simulink model "A2_SMART_Traffic_Automation_System_Outcome1"  (R2024b)
settings: Solver=VariableStepAuto  StartTime=0.0  StopTime=inf  RelTol=1e-3
settings Model: NumberOfSteps=2  Creator=User  LastModifiedBy=User

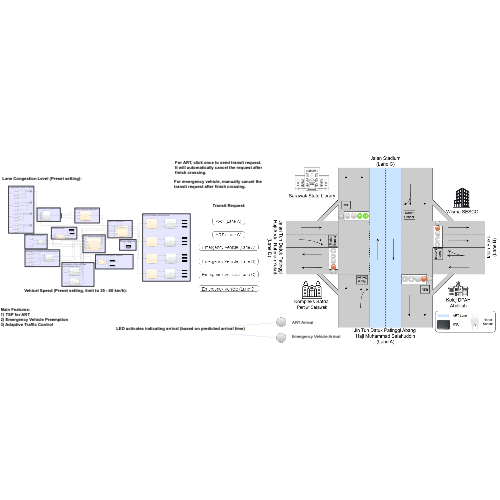
[thumbnail: Simulink's stored preview of the top-level diagram]
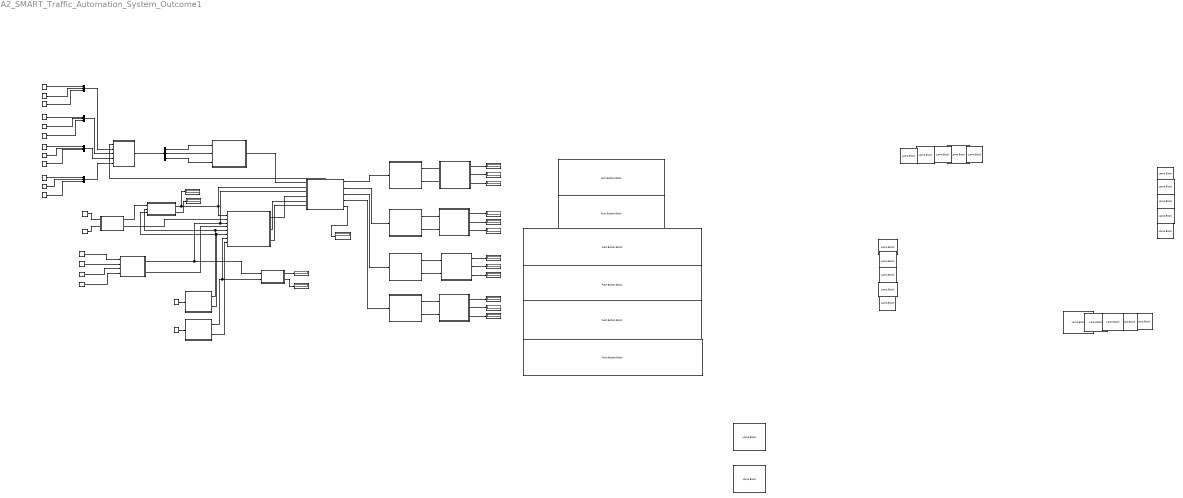
== system A2_SMART_Traffic_Automation_System_Outcome1 ==
  note: Transit Request:
  note: Lane A
  note: Congestion Level of Lanes
  note: Classification of Congestion Level
  note: Green Interval Selection
  note: Traffic Controller
  note: ART Transit Request
  note: Emergency Vehicle Transit Request
  note: Arrival of ART
  note: TSP Request Handling
  note: Arrival of Emergency Vehicle
  note: Calculation of Arrival Time
      | and Crossing Time
  note: Flash Signal
  note: Light Controller and Decoder
  note: ART Arrival
  note: Emergency Vehicle Arrival
  note: Lane B
  note: Lane C
  note: Lane D
  note: For ART, click once to send transit request. It will automatically cancel the request after finish crossing.
      |
      | For emergency vehicle, manually cancel the transit request after finish crossing.
  note: LED activates indicating arrival (based on predicted arrival time)
  note: Lane Congestion Level (Preset setting):
  note: Main Features:
      | 1) TSP for ART
      | 2) Emergency Vehicle Preemption
      | 3) Adaptive Traffic Control
  note: Vehicel Speed (Preset setting, limit to 35 - 80 km/h):
  ART Arrival : Display
  ART Transit Request : Display
  Calculation of ART Arrival Time and Crossing Time : Subsystem
  Calculation of Emergency Vehicle Arrival Time and Crossing Time : Subsystem
  Chart : Stateflow chart  TreatAsAtomicUnit=on
      settings: PortSchema="{\"entries\":[{\"content\":{\"sides\":[{\"content\":{\"connectorIds\":[\"In6\",\"In8\",\"In5\",\"In7\",\"In1\",\"In3\",\"In2\",\"In4\"]},\"type\":\"ConnectorPlacement.EquallySpacedRectSide\",\"uuid\":\"3b8b5f25-9f42-4404-a7ab-9a14576ba9bc\"},{\"content\":{\"connectorIds\":[\"Out3\",\"Out1\",\"Out2\"],\"side\":\"RIGHT\"},\"type\":\"ConnectorPlacement.EquallySpacedRectSide\",\"uuid\":\"4c53b1e2-c9f4-4e0d-a7f8-e259704f49e5\"},{\"content\":{\"side\":\"TOP\"},\"type\":\"ConnectorPlacement.EquallySpacedRectSide\",\"uuid\":\"8c5bac8d-90e8-4795-8438-ca30e0de2823\"}]},\"type\":\"ConnectorPlacement.EquallySpacedConnector\",\"uuid\":\"481cd6a2-dbd3-4912-a805-bd25a54799f5\"}],\"packageUris\":[\"http://schema.mathworks.com/mf0/Connector/R2020b\"],\"version\":\"1.0\"}"
  Chart1 : Stateflow chart  TreatAsAtomicUnit=on
  Chart2 : Stateflow chart  TreatAsAtomicUnit=on
      settings: PortSchema="{\"entries\":[{\"content\":{\"sides\":[{\"content\":{\"connectorIds\":[\"In1\",\"In2\"]},\"type\":\"ConnectorPlacement.EquallySpacedRectSide\",\"uuid\":\"14131ada-69d8-4c61-8553-b2a1dbc3d743\"},{\"content\":{\"connectorIds\":[\"Out2\",\"Out1\"],\"side\":\"RIGHT\"},\"type\":\"ConnectorPlacement.EquallySpacedRectSide\",\"uuid\":\"91a87b04-e272-4077-aa78-32a12e8e289e\"},{\"content\":{\"side\":\"TOP\"},\"type\":\"ConnectorPlacement.EquallySpacedRectSide\",\"uuid\":\"3c65f825-8df3-4d64-be65-7907849d7437\"}]},\"type\":\"ConnectorPlacement.EquallySpacedConnector\",\"uuid\":\"a2eb85a8-e87b-481d-83e5-614a6250d93d\"}],\"packageUris\":[\"http://schema.mathworks.com/mf0/Connector/R2020b\"],\"version\":\"1.0\"}"
  Decoder (Lane A) : Subsystem
  Decoder (Lane B) : Subsystem
  Decoder (Lane C) : Subsystem
  Decoder (Lane D) : Subsystem
  Demux : Demux  Outputs=3
  Display{,1..11} (12 alike) : Display
  Emergency Vehicle Arrival : Display
  Emergency Vehicle Transit Request : Display
  Flash : Display
  High Congestion A : Constant  Value=0
  High Congestion B : Constant  Value=0
  High Congestion C : Constant
  High Congestion D : Constant  Value=0
  Lamp{,1,12,16..17,20..23,26..27,29,31..32} (14 alike) : LampBlock  LabelPosition=Hide
  Lamp13 : LampBlock  LabelPosition=Hide  Icon=Custom  CustomIcon=data:image/svg+xml;base64,PD94bWwgdmVyc2lvbj0iMS4wIiBlbmNvZGluZz0idXRmLTgiPz4NCg0KPCEtLSBVcGxvYWRlZCB0bzogU1ZHIFJlcG8sIHd3dy5zdmdyZXBvLmNvbSwgR2VuZXJhdG9yOiBTVkcgUmVwbyBNaXhlciBUb29scyAtLT4KPHN2ZyBmaWxsPSIjMDAwMDAwIiBoZWlnaHQ9IjgwMHB4IiB3aWR0aD0iODAwcHgiIHZlcnNpb249IjEuMSIgaWQ9Ikljb25zIiB4bWxucz0iaHR0cDovL3d3dy53My5vcmcvMjAwMC9zdmciIHhtbG5zOnhsaW5rPSJodHRwOi8vd3d3LnczLm9yZy8xOTk5L3hsaW5rIiANCgkgdmlld0JveD0iMCAwIDMyIDMyIiB4bWw6c3BhY2U9InByZXNlcnZlIj4NCjxwYXRoIGQ9Ik0xNiwyQzguMywyLDIsOC4zLDIsMTZzNi4zLDE0LDE0LDE0czE0LTYuMywxNC0xNFMyMy43LDIsMTYsMnogTTIwLjcsMTUuN0MyMC41LDE1LjksMjAuMywxNiwyMCwxNnMtMC41LTAuMS0wLjctMC4zDQoJTDE3LDEzLjRWMjJjMCwwLjYtMC40LDEtMSwxcy0xLTAuNC0xLTF2LTguNmwtMi4zLDIuM2MtMC40LDAuNC0xLDAuNC0xLjQsMHMtMC40LTEsMC0xLjRsNC00YzAuMS0wLjEsMC4yLTAuMiwwLjMtMC4yDQoJYzAuMi0wLjEsMC41LTAuMSwwLjgsMGMwLjEsMC4xLDAuMiwwLjEsMC4zLDAuMmw0LDRDMjEuMSwxNC43LDIxLjEsMTUuMywyMC43LDE1Ljd6Ii8+DQo8L3N2Zz4=
  Lamp14 : LampBlock  LabelPosition=Hide  Icon=Custom  CustomIcon=data:image/svg+xml;base64,PD94bWwgdmVyc2lvbj0iMS4wIiBlbmNvZGluZz0iaXNvLTg4NTktMSI/Pg0KPCEtLSBVcGxvYWRlZCB0bzogU1ZHIFJlcG8sIHd3dy5zdmdyZXBvLmNvbSwgR2VuZXJhdG9yOiBTVkcgUmVwbyBNaXhlciBUb29scyAtLT4NCjxzdmcgaGVpZ2h0PSI4MDBweCIgd2lkdGg9IjgwMHB4IiB2ZXJzaW9uPSIxLjEiIGlkPSJDYXBhXzEiIHhtbG5zPSJodHRwOi8vd3d3LnczLm9yZy8yMDAwL3N2ZyIgeG1sbnM6eGxpbms9Imh0dHA6Ly93d3cudzMub3JnLzE5OTkveGxpbmsiIA0KCSB2aWV3Qm94PSIwIDAgMjYuOTI3IDI2LjkyNyIgeG1sOnNwYWNlPSJwcmVzZXJ2ZSI+DQo8Zz4NCgk8ZyBpZD0iYzE5NF9hcnJvdyI+DQoJCTxwYXRoIHN0eWxlPSJmaWxsOiMwMzAxMDQ7IiBkPSJNMTMuNDY0LDAuMDAyQzYuMDI3LDAuMDAyLDAsNi4wMjcsMCwxMy40NjRjMCw3LjQzNSw2LjAyNywxMy40NjIsMTMuNDY0LDEzLjQ2Mg0KCQkJYzcuNDMyLDAsMTMuNDYzLTYuMDI3LDEzLjQ2My0xMy40NjJDMjYuOTI4LDYuMDI3LDIwLjg5NiwwLjAwMiwxMy40NjQsMC4wMDJ6IE0yMi44MTYsMTUuMzAybC02LjM1NSw2LjM1NA0KCQkJYy0wLjgyNiwwLjgyOC0yLjEyMSwwLjg2Ny0yLjg5NSwwLjA5NGMtMC43NzItMC43NzMtMC43MzItMi4wNjgsMC4wOTQtMi44OTNsMy4wNC0zLjA0Mkg1LjQ0N2MtMS4wOTcsMC0xLjk4Mi0wLjg4OC0xLjk4NC0xLjk4MQ0KCQkJYzAtMS4wOTQsMC44ODctMS45OCwxLjk4NC0xLjk4aDExLjMxMUwxMy43MDIsOC44Yy0wLjgxMi0wLjgxNC0wLjg0Ny0yLjEwMy0wLjA3LTIuODc1YzAuNzczLTAuNzcyLDIuMDU4LTAuNzQxLDIuODcxLDAuMDczDQoJCQlsNi4yNzEsNi4yNjhjMC4wMjcsMC4wMjcsMC4wNDcsMC4wNjIsMC4wNywwLjA4OGMwLjAyMywwLjAyLDAuMDQ3LDAuMDMzLDAuMDY2LDAuMDU0QzIzLjY4NCwxMy4xNzcsMjMuNjQzLDE0LjQ3NCwyMi44MTYsMTUuMzAyeg0KCQkJIi8+DQoJPC9nPg0KPC9nPg0KPC9zdmc+
  Lamp18 : LampBlock  LabelPosition=Hide  Icon=Custom  CustomIcon=data:image/svg+xml;base64,PD94bWwgdmVyc2lvbj0iMS4wIiBlbmNvZGluZz0iVVRGLTgiIHN0YW5kYWxvbmU9Im5vIj8+DQo8IS0tIFVwbG9hZGVkIHRvOiBTVkcgUmVwbywgd3d3LnN2Z3JlcG8uY29tLCBHZW5lcmF0b3I6IFNWRyBSZXBvIE1peGVyIFRvb2xzIC0tPg0KPHN2ZyB3aWR0aD0iODAwcHgiIGhlaWdodD0iODAwcHgiIHZpZXdCb3g9IjAgMCAzMiAzMiIgdmVyc2lvbj0iMS4xIiB4bWxucz0iaHR0cDovL3d3dy53My5vcmcvMjAwMC9zdmciIHhtbG5zOnhsaW5rPSJodHRwOi8vd3d3LnczLm9yZy8xOTk5L3hsaW5rIiB4bWxuczpza2V0Y2g9Imh0dHA6Ly93d3cuYm9oZW1pYW5jb2RpbmcuY29tL3NrZXRjaC9ucyI+DQogICAgDQogICAgPHRpdGxlPmFycm93LXJpZ2h0LWNpcmNsZTwvdGl0bGU+DQogICAgPGRlc2M+Q3JlYXRlZCB3aXRoIFNrZXRjaCBCZXRhLjwvZGVzYz4NCiAgICA8ZGVmcz4NCg0KPC9kZWZzPg0KICAgIDxnIGlkPSJQYWdlLTEiIHN0cm9rZT0ibm9uZSIgc3Ryb2tlLXdpZHRoPSIxIiBmaWxsPSJub25lIiBmaWxsLXJ1bGU9ImV2ZW5vZGQiIHNrZXRjaDp0eXBlPSJNU1BhZ2UiPg0KICAgICAgICA8ZyBpZD0iSWNvbi1TZXQtRmlsbGVkIiBza2V0Y2g6dHlwZT0iTVNMYXllckdyb3VwIiB0cmFuc2Zvcm09InRyYW5zbGF0ZSgtMzEwLjAwMDAwMCwgLTEwODkuMDAwMDAwKSIgZmlsbD0iIzAwMDAwMCI+DQogICAgICAgICAgICA8cGF0aCBkPSJNMzMyLjUzNSwxMTA1Ljg4IEwzMjYuODc5LDExMTEuNTQgQzMyNi40ODgsMTExMS45MyAzMjUuODU1LDExMTEuOTMgMzI1LjQ2NSwxMTExLjU0IEMzMjUuMDc0LDExMTEuMTUgMzI1LjA3NCwxMTEwLjUxIDMyNS40NjUsMTExMC4xMiBMMzI5LjU4NiwxMTA2IEwzMTksMTEwNiBDMzE4LjQ0NywxMTA2IDMxOCwxMTA1LjU1IDMxOCwxMTA1IEMzMTgsMTEwNC40NSAzMTguNDQ3LDExMDQgMzE5LDExMDQgTDMyOS41ODYsMTEwNCBMMzI1LjQ2NSwxMDk5Ljg4IEMzMjUuMDc0LDEwOTkuNDkgMzI1LjA3NCwxMDk4Ljg2IDMyNS40NjUsMTA5OC40NiBDMzI1Ljg1NSwxMDk4LjA3IDMyNi40ODgsMTA5OC4wNyAzMjYuODc5LDEwOTguNDYgTDMzMi41MzUsMTEwNC4xMiBDMzMyLjc3NSwxMTA0LjM2IDMzMi44NSwxMTA0LjY5IDMzMi43OTUsMTEwNSBDMzMyLjg1LDExMDUuMzEgMzMyLjc3NSwxMTA1LjY0IDMzMi41MzUsMTEwNS44OCBMMzMyLjUzNSwxMTA1Ljg4IFogTTMyNiwxMDg5IEMzMTcuMTYzLDEwODkgMzEwLDEwOTYuMTYgMzEwLDExMDUgQzMxMCwxMTEzLjg0IDMxNy4xNjMsMTEyMSAzMjYsMTEyMSBDMzM0LjgzNywxMTIxIDM0MiwxMTEzLjg0IDM0MiwxMTA1IEMzNDIsMTA5Ni4xNiAzMzQuODM3LDEwODkgMzI2LDEwODkgTDMyNiwxMDg5IFoiIGlkPSJhcnJvdy1yaWdodC1jaXJjbGUiIHNrZXRjaDp0eXBlPSJNU1NoYXBlR3JvdXAiPg0KDQo8L3BhdGg+DQogICAgICAgIDwvZz4NCiAgICA8L2c+DQo8L3N2Zz4=
  Lamp19 : LampBlock  LabelPosition=Hide  Icon=Custom  CustomIcon=data:image/svg+xml;base64,PD94bWwgdmVyc2lvbj0iMS4wIiBlbmNvZGluZz0idXRmLTgiPz4KDTwhLS0gVXBsb2FkZWQgdG86IFNWRyBSZXBvLCB3d3cuc3ZncmVwby5jb20sIEdlbmVyYXRvcjogU1ZHIFJlcG8gTWl4ZXIgVG9vbHMgLS0+Cjxzdmcgd2lkdGg9IjgwMHB4IiBoZWlnaHQ9IjgwMHB4IiB2aWV3Qm94PSIwIDAgMjQgMjQiIHhtbG5zPSJodHRwOi8vd3d3LnczLm9yZy8yMDAwL3N2ZyI+CiAgICA8Zz4KICAgICAgICA8cGF0aCBmaWxsPSJub25lIiBkPSJNMCAwaDI0djI0SDB6Ii8+CiAgICAgICAgPHBhdGggZD0iTTEyIDJjNS41MiAwIDEwIDQuNDggMTAgMTBzLTQuNDggMTAtMTAgMTBTMiAxNy41MiAyIDEyIDYuNDggMiAxMiAyem0wIDlWOGwtNCA0IDQgNHYtM2g0di0yaC00eiIvPgogICAgPC9nPgo8L3N2Zz4=
  Lamp24 : LampBlock  LabelPosition=Hide  Icon=Custom  CustomIcon=data:image/svg+xml;base64,PD94bWwgdmVyc2lvbj0iMS4wIiBlbmNvZGluZz0iaXNvLTg4NTktMSI/Pg0KPCEtLSBVcGxvYWRlZCB0bzogU1ZHIFJlcG8sIHd3dy5zdmdyZXBvLmNvbSwgR2VuZXJhdG9yOiBTVkcgUmVwbyBNaXhlciBUb29scyAtLT4NCjwhRE9DVFlQRSBzdmcgUFVCTElDICItLy9XM0MvL0RURCBTVkcgMS4xLy9FTiIgImh0dHA6Ly93d3cudzMub3JnL0dyYXBoaWNzL1NWRy8xLjEvRFREL3N2ZzExLmR0ZCI+DQo8c3ZnIGZpbGw9IiMwMDAwMDAiIHZlcnNpb249IjEuMSIgaWQ9IkNhcGFfMSIgeG1sbnM9Imh0dHA6Ly93d3cudzMub3JnLzIwMDAvc3ZnIiB4bWxuczp4bGluaz0iaHR0cDovL3d3dy53My5vcmcvMTk5OS94bGluayIgDQoJIHdpZHRoPSI4MDBweCIgaGVpZ2h0PSI4MDBweCIgdmlld0JveD0iMCAwIDQwIDQwIiB4bWw6c3BhY2U9InByZXNlcnZlIj4NCjxnPg0KCTxwYXRoIGQ9Ik0yMCwwQzguOTczLDAsMCw4Ljk3MywwLDIwYzAsMTEuMDI3LDguOTczLDIwLDIwLDIwYzExLjAyNywwLDIwLTguOTczLDIwLTIwQzQwLDguOTczLDMxLjAyNywwLDIwLDB6IE0yOC4wMTgsMTkuNzUyDQoJCWMtMC40NTEsMC41MzEtMS4wOTQsMC44MDUtMS43MzgsMC44MDVjLTAuNTIxLDAtMS4wNDctMC4xNzktMS40NzctMC41NDNsLTIuNTIxLTIuMTQxdjkuMTg2YzAsMS4yNi0xLjAyMSwyLjI4LTIuMjgxLDIuMjgNCgkJYy0xLjI2LDAtMi4yODEtMS4wMjEtMi4yODEtMi4yOHYtOS4xODZsLTIuNTIxLDIuMTQxYy0wLjk2LDAuODE2LTIuNCwwLjY5OC0zLjIxNi0wLjI2MmMtMC44MTYtMC45NjEtMC42OTgtMi40LDAuMjYyLTMuMjE2DQoJCWw2LjI3OS01LjMzM2MwLjg1Mi0wLjcyMywyLjEwMi0wLjcyMywyLjk1NSwwbDYuMjc4LDUuMzMzQzI4LjcxNiwxNy4zNTIsMjguODM0LDE4Ljc5MSwyOC4wMTgsMTkuNzUyeiIvPg0KPC9nPg0KPC9zdmc+
  Lamp25 : LampBlock  LabelPosition=Hide  Icon=Custom  CustomIcon=data:image/svg+xml;base64,PD94bWwgdmVyc2lvbj0iMS4wIiBlbmNvZGluZz0iaXNvLTg4NTktMSI/Pg0KPCEtLSBVcGxvYWRlZCB0bzogU1ZHIFJlcG8sIHd3dy5zdmdyZXBvLmNvbSwgR2VuZXJhdG9yOiBTVkcgUmVwbyBNaXhlciBUb29scyAtLT4NCjwhRE9DVFlQRSBzdmcgUFVCTElDICItLy9XM0MvL0RURCBTVkcgMS4xLy9FTiIgImh0dHA6Ly93d3cudzMub3JnL0dyYXBoaWNzL1NWRy8xLjEvRFREL3N2ZzExLmR0ZCI+DQo8c3ZnIGZpbGw9IiMwMDAwMDAiIHZlcnNpb249IjEuMSIgaWQ9IkNhcGFfMSIgeG1sbnM9Imh0dHA6Ly93d3cudzMub3JnLzIwMDAvc3ZnIiB4bWxuczp4bGluaz0iaHR0cDovL3d3dy53My5vcmcvMTk5OS94bGluayIgDQoJIHdpZHRoPSI4MDBweCIgaGVpZ2h0PSI4MDBweCIgdmlld0JveD0iMCAwIDQwIDQwIiB4bWw6c3BhY2U9InByZXNlcnZlIj4NCjxnPg0KCTxwYXRoIGQ9Ik0yMCwwQzguOTczLDAsMCw4Ljk3MywwLDIwYzAsMTEuMDI3LDguOTczLDIwLDIwLDIwYzExLjAyNywwLDIwLTguOTczLDIwLTIwQzQwLDguOTczLDMxLjAyNywwLDIwLDB6IE0yNy43NTYsMjMuNDY1DQoJCWwtNi4yNzksNS4zMzJDMjEuMDUxLDI5LjE1OCwyMC41MjUsMjkuMzQsMjAsMjkuMzRjLTAuNTI2LDAtMS4wNTItMC4xODItMS40NzgtMC41NDNsLTYuMjc5LTUuMzMyDQoJCWMtMC45NTktMC44MTYtMS4wNzctMi4yNTYtMC4yNjItMy4yMTdjMC44MTUtMC45NTksMi4yNTUtMS4wNzgsMy4yMTYtMC4yNjJsMi41MjEsMi4xNDF2LTkuMTg2YzAtMS4yNiwxLjAyMS0yLjI4MSwyLjI4Mi0yLjI4MQ0KCQljMS4yNiwwLDIuMjgxLDEuMDIxLDIuMjgxLDIuMjgxdjkuMTg2bDIuNTIxLTIuMTQxYzAuOTYyLTAuODE0LDIuNDAxLTAuNjk3LDMuMjE4LDAuMjYyDQoJCUMyOC44MzQsMjEuMjA5LDI4LjcxNiwyMi42NDgsMjcuNzU2LDIzLjQ2NXoiLz4NCjwvZz4NCjwvc3ZnPg==
  Lamp28 : LampBlock  LabelPosition=Hide  Icon=Custom  CustomIcon=data:image/svg+xml;base64,PD94bWwgdmVyc2lvbj0iMS4wIiBlbmNvZGluZz0idXRmLTgiPz4KDTwhLS0gVXBsb2FkZWQgdG86IFNWRyBSZXBvLCB3d3cuc3ZncmVwby5jb20sIEdlbmVyYXRvcjogU1ZHIFJlcG8gTWl4ZXIgVG9vbHMgLS0+Cjxzdmcgd2lkdGg9IjgwMHB4IiBoZWlnaHQ9IjgwMHB4IiB2aWV3Qm94PSIwIDAgMjQgMjQiIHhtbG5zPSJodHRwOi8vd3d3LnczLm9yZy8yMDAwL3N2ZyI+CiAgICA8Zz4KICAgICAgICA8cGF0aCBmaWxsPSJub25lIiBkPSJNMCAwaDI0djI0SDB6Ii8+CiAgICAgICAgPHBhdGggZD0iTTEyIDJjNS41MiAwIDEwIDQuNDggMTAgMTBzLTQuNDggMTAtMTAgMTBTMiAxNy41MiAyIDEyIDYuNDggMiAxMiAyem0wIDlWOGwtNCA0IDQgNHYtM2g0di0yaC00eiIvPgogICAgPC9nPgo8L3N2Zz4=
  Lamp30 : LampBlock  LabelPosition=Hide  Icon=Custom  CustomIcon=data:image/svg+xml;base64,PD94bWwgdmVyc2lvbj0iMS4wIiBlbmNvZGluZz0iaXNvLTg4NTktMSI/Pg0KPCEtLSBVcGxvYWRlZCB0bzogU1ZHIFJlcG8sIHd3dy5zdmdyZXBvLmNvbSwgR2VuZXJhdG9yOiBTVkcgUmVwbyBNaXhlciBUb29scyAtLT4NCjwhRE9DVFlQRSBzdmcgUFVCTElDICItLy9XM0MvL0RURCBTVkcgMS4xLy9FTiIgImh0dHA6Ly93d3cudzMub3JnL0dyYXBoaWNzL1NWRy8xLjEvRFREL3N2ZzExLmR0ZCI+DQo8c3ZnIGZpbGw9IiMwMDAwMDAiIHZlcnNpb249IjEuMSIgaWQ9IkNhcGFfMSIgeG1sbnM9Imh0dHA6Ly93d3cudzMub3JnLzIwMDAvc3ZnIiB4bWxuczp4bGluaz0iaHR0cDovL3d3dy53My5vcmcvMTk5OS94bGluayIgDQoJIHdpZHRoPSI4MDBweCIgaGVpZ2h0PSI4MDBweCIgdmlld0JveD0iMCAwIDQwIDQwIiB4bWw6c3BhY2U9InByZXNlcnZlIj4NCjxnPg0KCTxwYXRoIGQ9Ik0yMCwwQzguOTczLDAsMCw4Ljk3MywwLDIwYzAsMTEuMDI3LDguOTczLDIwLDIwLDIwYzExLjAyNywwLDIwLTguOTczLDIwLTIwQzQwLDguOTczLDMxLjAyNywwLDIwLDB6IE0yNy43NTYsMjMuNDY1DQoJCWwtNi4yNzksNS4zMzJDMjEuMDUxLDI5LjE1OCwyMC41MjUsMjkuMzQsMjAsMjkuMzRjLTAuNTI2LDAtMS4wNTItMC4xODItMS40NzgtMC41NDNsLTYuMjc5LTUuMzMyDQoJCWMtMC45NTktMC44MTYtMS4wNzctMi4yNTYtMC4yNjItMy4yMTdjMC44MTUtMC45NTksMi4yNTUtMS4wNzgsMy4yMTYtMC4yNjJsMi41MjEsMi4xNDF2LTkuMTg2YzAtMS4yNiwxLjAyMS0yLjI4MSwyLjI4Mi0yLjI4MQ0KCQljMS4yNiwwLDIuMjgxLDEuMDIxLDIuMjgxLDIuMjgxdjkuMTg2bDIuNTIxLTIuMTQxYzAuOTYyLTAuODE0LDIuNDAxLTAuNjk3LDMuMjE4LDAuMjYyDQoJCUMyOC44MzQsMjEuMjA5LDI4LjcxNiwyMi42NDgsMjcuNzU2LDIzLjQ2NXoiLz4NCjwvZz4NCjwvc3ZnPg==
  Lane A (ART) : Constant  Value=0
  Lane A (Emergency Vehicle) : Constant  Value=0
  Lane B (Emergency Vehicle) : Constant  Value=0
  Lane C (ART) : Constant  Value=0
  Lane C (Emergency Vehicle) : Constant  Value=0
  Lane D (Emergency Vehicle) : Constant  Value=0
  Light Controller (A) : Stateflow chart  TreatAsAtomicUnit=on
  Light Controller (B) : Stateflow chart  TreatAsAtomicUnit=on
  Light Controller (C) : Stateflow chart  TreatAsAtomicUnit=on
  Light Controller (D) : Stateflow chart  TreatAsAtomicUnit=on
  Low Congestion A : Constant
  Low Congestion B : Constant  Value=0
  Low Congestion C : Constant  Value=0
  Low Congestion D : Constant
  Medium Congestion A : Constant  Value=0
  Medium Congestion B : Constant
  Medium Congestion C : Constant  Value=0
  Medium Congestion D : Constant  Value=0
  Mux{,1..3} (4 alike) : Mux  Inputs=3
  Push Button : PushButtonBlock  ButtonText=ART (Lane A)  OffValue=0.000000
  Push Button1 : PushButtonBlock  ButtonText=ART (Lane C)  OffValue=0.000000
  Push Button2 : PushButtonBlock  ButtonText=Emergency Vehicle (Lane A)  ButtonType=Latch  OffValue=0.000000
  Push Button3 : PushButtonBlock  ButtonText=Emergency Vehicle (Lane B)  ButtonType=Latch  OffValue=0.000000
  Push Button4 : PushButtonBlock  ButtonText=Emergency Vehicle (Lane C)  ButtonType=Latch  OffValue=0.000000
  Push Button5 : PushButtonBlock  ButtonText=Emergency Vehicle (Lane D)  ButtonType=Latch  OffValue=0.000000
  Speed (km/h) : Constant  Value=60
  Speed (km/h)1 : Constant  Value=40
  Subsystem : Subsystem
  Subsystem1 : Subsystem
  Subsystem2 : Subsystem
  Traffic Congestion Determination : Stateflow chart  TreatAsAtomicUnit=on
  Trafftc Controller : Stateflow chart  TreatAsAtomicUnit=on
      settings: PortSchema="{\"entries\":[{\"content\":{\"sides\":[{\"content\":{\"connectorIds\":[\"In1\",\"In4\",\"In5\",\"In6\",\"In2\",\"In3\"]},\"type\":\"ConnectorPlacement.EquallySpacedRectSide\",\"uuid\":\"8dd1b2e6-86fe-49ce-8a55-3d5fe398c3d7\"},{\"content\":{\"connectorIds\":[\"Out1\",\"Out2\",\"Out3\",\"Out4\",\"Out5\"],\"side\":\"RIGHT\"},\"type\":\"ConnectorPlacement.EquallySpacedRectSide\",\"uuid\":\"2d2da7fc-60fb-456f-9fa8-4a212ac68bd8\"},{\"content\":{\"connectorIds\":[\"Out6\"],\"side\":\"TOP\"},\"type\":\"ConnectorPlacement.EquallySpacedRectSide\",\"uuid\":\"d96f078d-ebed-48bc-8cec-384ff6a47410\"}]},\"type\":\"ConnectorPlacement.EquallySpacedConnector\",\"uuid\":\"06e33d01-c1fa-4305-8173-8a90a3d39650\"}],\"packageUris\":[\"http://schema.mathworks.com/mf0/Connector/R2020b\"],\"version\":\"1.0\"}"
  wires:
  Light Controller (A)/1(S0) -> Decoder (Lane A)/1(S0)
  Light Controller (C)/1(S0) -> Decoder (Lane C)/1(S0)
  Trafftc Controller/1(A) -> Light Controller (A)/1(Green)
  Decoder (Lane D)/2(Green) -> Display10/1
  Light Controller (C)/2(S1) -> Decoder (Lane C)/2(S1)
  Decoder (Lane A)/1(Red) -> Display/1
  Decoder (Lane D)/1(Red) -> Display9/1
  Light Controller (B)/1(S0) -> Decoder (Lane B)/1(S0)
  Decoder (Lane C)/1(Red) -> Display3/1
  Decoder (Lane C)/3(Amber) -> Display8/1
  Trafftc Controller/2(B) -> Light Controller (B)/1(Green)
  Light Controller (D)/1(S0) -> Decoder (Lane D)/1(S0)
  Trafftc Controller/4(D) -> Light Controller (D)/1(Green)
  Decoder (Lane A)/3(Amber) -> Display2/1
  Trafftc Controller/3(C) -> Light Controller (C)/1(Green)
  Decoder (Lane D)/3(Amber) -> Display11/1
  Decoder (Lane A)/2(Green) -> Display1/1
  Light Controller (D)/2(S1) -> Decoder (Lane D)/2(S1)
  Light Controller (A)/2(S1) -> Decoder (Lane A)/2(S1)
  Decoder (Lane B)/3(Amber) -> Display6/1
  Decoder (Lane B)/2(Green) -> Display5/1
  Decoder (Lane C)/2(Green) -> Display7/1
  Decoder (Lane B)/1(Red) -> Display4/1
  Light Controller (B)/2(S1) -> Decoder (Lane B)/2(S1)
  Trafftc Controller/5(Flash) -> Flash/1
  Speed (km/h)/1 -> Calculation of ART Arrival Time and Crossing Time/1(Speed)
  Chart/1(ArrivalTime) -> Trafftc Controller/2(ArrivalTime)
  Chart/2(CrossingTime) -> Trafftc Controller/3(CrossingTime)
  Chart/3(At) -> Trafftc Controller/6(At)
  Speed (km/h)1/1 -> Calculation of Emergency Vehicle Arrival Time and Crossing Time/1(Speed)
  Calculation of ART Arrival Time and Crossing Time/1(ArrivalTime) -> Chart1/2(ArrivalTime), Chart/1(ArrivalTime_ART)
  Calculation of ART Arrival Time and Crossing Time/2(CrossingTime) -> Chart1/3(CrossingTime), Chart/3(CrossingTime_ART)
  Calculation of Emergency Vehicle Arrival Time and Crossing Time/1(ArrivalTime) -> Chart/2(ArrivalTime_Emergency), Chart2/2(ArrivalTime)
  Calculation of Emergency Vehicle Arrival Time and Crossing Time/2(CrossingTime) -> Chart/4(CrossingTime_Emergency)
  Traffic Congestion Determination/1(GreenInterval) -> Trafftc Controller/1(GreenInterval)
  Lane A (ART)/1 -> Subsystem/1(Lane A)
  Lane C (ART)/1 -> Subsystem/2(Lane C)
  Subsystem/2(ART location) -> Chart/8(At_ART)
  Lane B (Emergency Vehicle)/1 -> Subsystem2/2(Lane B)
  Lane A (Emergency Vehicle)/1 -> Subsystem2/1(Lane A)
  Lane C (Emergency Vehicle)/1 -> Subsystem2/3(Lane C)
  Lane D (Emergency Vehicle)/1 -> Subsystem2/4(Lane D)
  Subsystem2/2(Emergency Vehicle location) -> Chart/7(At_Emergency)
  Medium Congestion A/1 -> Mux/2
  Low Congestion A/1 -> Mux/1
  High Congestion A/1 -> Mux/3
  Low Congestion B/1 -> Mux1/1
  Medium Congestion B/1 -> Mux1/2
  High Congestion B/1 -> Mux1/3
  Low Congestion C/1 -> Mux2/1
  Medium Congestion C/1 -> Mux2/2
  High Congestion C/1 -> Mux2/3
  High Congestion D/1 -> Mux3/3
  Low Congestion D/1 -> Mux3/1
  Medium Congestion D/1 -> Mux3/2
  Mux/1 -> Subsystem1/2(In2)
  Mux1/1 -> Subsystem1/3(In3)
  Mux2/1 -> Subsystem1/4(In4)
  Mux3/1 -> Subsystem1/5(In5)
  Trafftc Controller/6(PrevLane) -> Subsystem1/1(PrevLane)
  Subsystem1/1(Out1) -> Demux/1
  Demux/1 -> Traffic Congestion Determination/1(Low)
  Demux/2 -> Traffic Congestion Determination/2(Medium)
  Demux/3 -> Traffic Congestion Determination/3(High)
  Subsystem/1(TSP Request) -> Chart1/1(TSP)
  Chart1/1(ART) -> Trafftc Controller/4(ART), Chart/6(ART), ART Transit Request/1
  Subsystem2/1(TSP Request) -> Chart2/1(TSP), Trafftc Controller/5(Emergency), Chart/5(Emergency)
  Chart1/2(Arrived) -> ART Arrival/1
  Chart2/2(Emergency) -> Emergency Vehicle Transit Request/1
  Chart2/1(Arrived) -> Emergency Vehicle Arrival/1

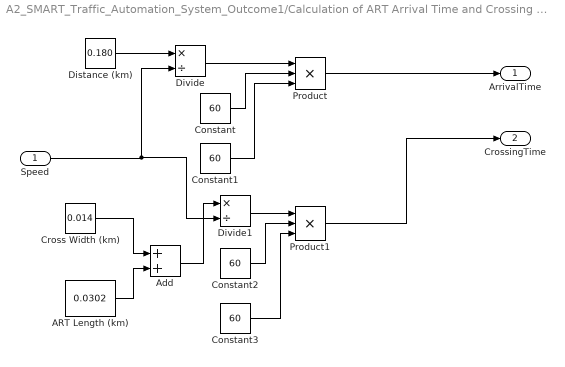
== system A2_SMART_Traffic_Automation_System_Outcome1/Calculation of ART Arrival Time and Crossing Time ==
  Speed : Inport
  ART Length (km) : Constant  Value=0.0302
  Add : Sum
  Constant{,1..3} (4 alike) : Constant  Value=60
  Cross Width (km) : Constant  Value=0.014
  Distance (km) : Constant  Value=0.180
  Divide : Product  Inputs=*/
  Divide1 : Product  Inputs=*/
  Product : Product  Inputs=3
  Product1 : Product  Inputs=3
  ArrivalTime : Outport
  CrossingTime : Outport  Port=2
  wires:
  Speed/1 -> Divide/2, Divide1/2
  Divide/1 -> Product/1
  Distance (km)/1 -> Divide/1
  Constant/1 -> Product/2
  Divide1/1 -> Product1/1
  Constant1/1 -> Product/3
  Product1/1 -> CrossingTime/1
  Product/1 -> ArrivalTime/1
  ART Length (km)/1 -> Add/2
  Cross Width (km)/1 -> Add/1
  Add/1 -> Divide1/1
  Constant2/1 -> Product1/2
  Constant3/1 -> Product1/3

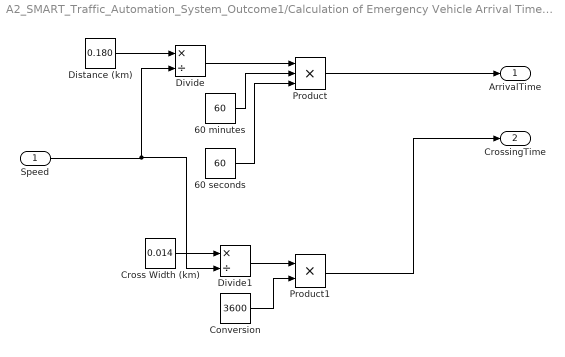
== system A2_SMART_Traffic_Automation_System_Outcome1/Calculation of Emergency Vehicle Arrival Time and Crossing Time ==
  Speed : Inport
  60 minutes : Constant  Value=60
  60 seconds : Constant  Value=60
  Conversion : Constant  Value=3600
  Cross Width (km) : Constant  Value=0.014
  Distance (km) : Constant  Value=0.180
  Divide : Product  Inputs=*/
  Divide1 : Product  Inputs=*/
  Product : Product  Inputs=3
  Product1 : Product
  ArrivalTime : Outport
  CrossingTime : Outport  Port=2
  wires:
  Conversion/1 -> Product1/2
  Speed/1 -> Divide/2, Divide1/2
  Divide/1 -> Product/1
  Distance (km)/1 -> Divide/1
  60 minutes/1 -> Product/2
  Cross Width (km)/1 -> Divide1/1
  Divide1/1 -> Product1/1
  60 seconds/1 -> Product/3
  Product1/1 -> CrossingTime/1
  Product/1 -> ArrivalTime/1

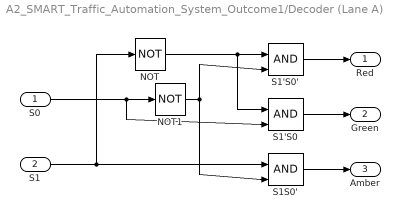
== system A2_SMART_Traffic_Automation_System_Outcome1/Decoder (Lane A) ==
  S0 : Inport
  S1 : Inport  Port=2
  NOT : Logic  Operator=NOT  IconShape=distinctive  AllPortsSameDT=off  OutDataTypeStr=boolean
  NOT1 : Logic  Operator=NOT  IconShape=distinctive  AllPortsSameDT=off  OutDataTypeStr=boolean
  S1'S0 : Logic  IconShape=distinctive  AllPortsSameDT=off  OutDataTypeStr=boolean
  S1'S0' : Logic  IconShape=distinctive  AllPortsSameDT=off  OutDataTypeStr=boolean
  S1S0' : Logic  IconShape=distinctive  AllPortsSameDT=off  OutDataTypeStr=boolean
  Red : Outport
  Green : Outport  Port=2
  Amber : Outport  Port=3
  wires:
  S0/1 -> S1'S0/2, NOT1/1
  NOT1/1 -> S1S0'/2, S1'S0'/2
  NOT/1 -> S1'S0'/1, S1'S0/1
  S1/1 -> NOT/1, S1S0'/1
  S1'S0/1 -> Green/1
  S1S0'/1 -> Amber/1
  S1'S0'/1 -> Red/1

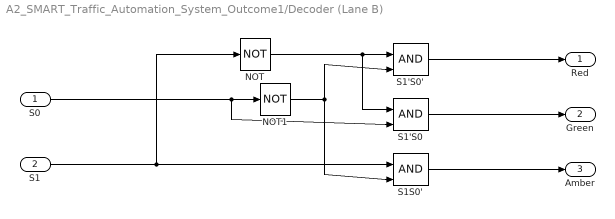
== system A2_SMART_Traffic_Automation_System_Outcome1/Decoder (Lane B) ==
  S0 : Inport
  S1 : Inport  Port=2
  NOT : Logic  Operator=NOT  IconShape=distinctive  AllPortsSameDT=off  OutDataTypeStr=boolean
  NOT1 : Logic  Operator=NOT  IconShape=distinctive  AllPortsSameDT=off  OutDataTypeStr=boolean
  S1'S0 : Logic  IconShape=distinctive  AllPortsSameDT=off  OutDataTypeStr=boolean
  S1'S0' : Logic  IconShape=distinctive  AllPortsSameDT=off  OutDataTypeStr=boolean
  S1S0' : Logic  IconShape=distinctive  AllPortsSameDT=off  OutDataTypeStr=boolean
  Red : Outport
  Green : Outport  Port=2
  Amber : Outport  Port=3
  wires:
  S0/1 -> S1'S0/2, NOT1/1
  NOT1/1 -> S1S0'/2, S1'S0'/2
  NOT/1 -> S1'S0'/1, S1'S0/1
  S1/1 -> NOT/1, S1S0'/1
  S1'S0/1 -> Green/1
  S1S0'/1 -> Amber/1
  S1'S0'/1 -> Red/1

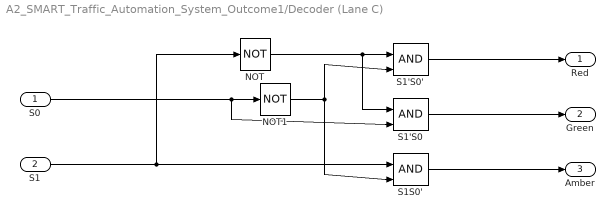
== system A2_SMART_Traffic_Automation_System_Outcome1/Decoder (Lane C) ==
  S0 : Inport
  S1 : Inport  Port=2
  NOT : Logic  Operator=NOT  IconShape=distinctive  AllPortsSameDT=off  OutDataTypeStr=boolean
  NOT1 : Logic  Operator=NOT  IconShape=distinctive  AllPortsSameDT=off  OutDataTypeStr=boolean
  S1'S0 : Logic  IconShape=distinctive  AllPortsSameDT=off  OutDataTypeStr=boolean
  S1'S0' : Logic  IconShape=distinctive  AllPortsSameDT=off  OutDataTypeStr=boolean
  S1S0' : Logic  IconShape=distinctive  AllPortsSameDT=off  OutDataTypeStr=boolean
  Red : Outport
  Green : Outport  Port=2
  Amber : Outport  Port=3
  wires:
  S0/1 -> S1'S0/2, NOT1/1
  NOT1/1 -> S1S0'/2, S1'S0'/2
  NOT/1 -> S1'S0'/1, S1'S0/1
  S1/1 -> NOT/1, S1S0'/1
  S1'S0/1 -> Green/1
  S1S0'/1 -> Amber/1
  S1'S0'/1 -> Red/1

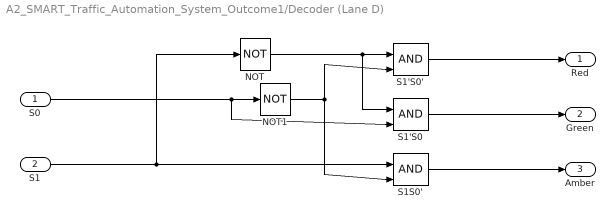
== system A2_SMART_Traffic_Automation_System_Outcome1/Decoder (Lane D) ==
  S0 : Inport
  S1 : Inport  Port=2
  NOT : Logic  Operator=NOT  IconShape=distinctive  AllPortsSameDT=off  OutDataTypeStr=boolean
  NOT1 : Logic  Operator=NOT  IconShape=distinctive  AllPortsSameDT=off  OutDataTypeStr=boolean
  S1'S0 : Logic  IconShape=distinctive  AllPortsSameDT=off  OutDataTypeStr=boolean
  S1'S0' : Logic  IconShape=distinctive  AllPortsSameDT=off  OutDataTypeStr=boolean
  S1S0' : Logic  IconShape=distinctive  AllPortsSameDT=off  OutDataTypeStr=boolean
  Red : Outport
  Green : Outport  Port=2
  Amber : Outport  Port=3
  wires:
  S0/1 -> S1'S0/2, NOT1/1
  NOT1/1 -> S1S0'/2, S1'S0'/2
  NOT/1 -> S1'S0'/1, S1'S0/1
  S1/1 -> NOT/1, S1S0'/1
  S1'S0/1 -> Green/1
  S1S0'/1 -> Amber/1
  S1'S0'/1 -> Red/1

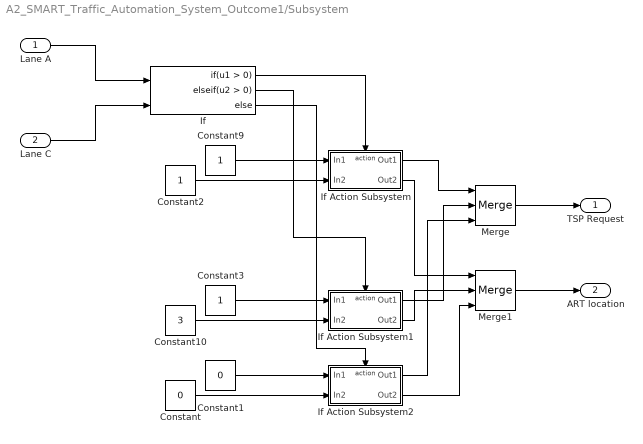
== system A2_SMART_Traffic_Automation_System_Outcome1/Subsystem ==
  Lane A : Inport
  Lane C : Inport  Port=2
  Constant : Constant  Value=0
  Constant1 : Constant  Value=0
  Constant10 : Constant  Value=3
  Constant2 : Constant
  Constant3 : Constant
  Constant9 : Constant
  If : If  NumInputs=2  ElseIfExpressions=u2 > 0
  If Action Subsystem : Subsystem  TreatAsAtomicUnit=on
  If Action Subsystem1 : Subsystem  TreatAsAtomicUnit=on
  If Action Subsystem2 : Subsystem  TreatAsAtomicUnit=on
  Merge : Merge  Inputs=3
  Merge1 : Merge  Inputs=3
  TSP Request : Outport
  ART location : Outport  Port=2
  wires:
  If/2 -> If Action Subsystem1/Action
  If/1 -> If Action Subsystem/Action
  If/3 -> If Action Subsystem2/Action
  Constant9/1 -> If Action Subsystem/1(In1)
  If Action Subsystem1/1(Out1) -> Merge/2
  If Action Subsystem/1(Out1) -> Merge/1
  Lane A/1 -> If/1
  Lane C/1 -> If/2
  Constant1/1 -> If Action Subsystem2/1(In1)
  If Action Subsystem2/1(Out1) -> Merge/3
  Constant2/1 -> If Action Subsystem/2(In2)
  Constant/1 -> If Action Subsystem2/2(In2)
  If Action Subsystem/2(Out2) -> Merge1/1
  If Action Subsystem1/2(Out2) -> Merge1/2
  If Action Subsystem2/2(Out2) -> Merge1/3
  Merge1/1 -> ART location/1
  Merge/1 -> TSP Request/1
  Constant10/1 -> If Action Subsystem1/2(In2)
  Constant3/1 -> If Action Subsystem1/1(In1)

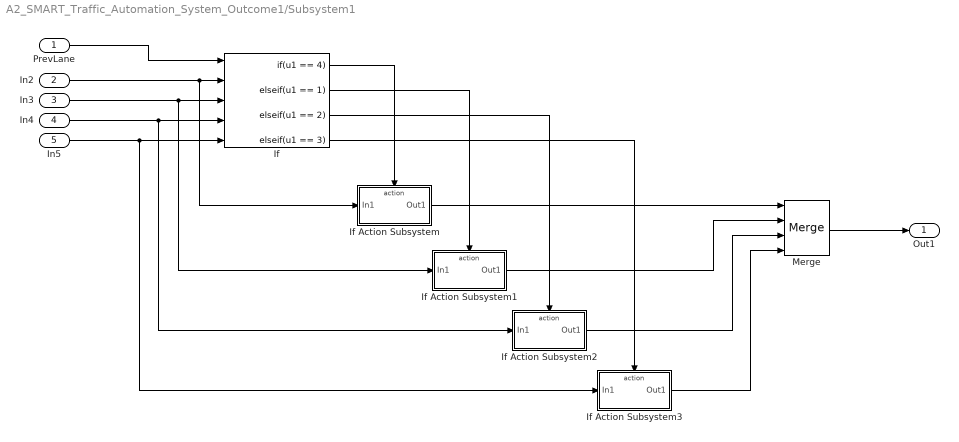
== system A2_SMART_Traffic_Automation_System_Outcome1/Subsystem1 ==
  PrevLane : Inport
  In2 : Inport  Port=2
  In3 : Inport  Port=3
  In4 : Inport  Port=4
  In5 : Inport  Port=5
  If : If  NumInputs=5  IfExpression=u1 == 4  ElseIfExpressions=u1 == 1, u1 == 2, u1 == 3  ShowElse=off
  If Action Subsystem : Subsystem  TreatAsAtomicUnit=on
  If Action Subsystem1 : Subsystem  TreatAsAtomicUnit=on
  If Action Subsystem2 : Subsystem  TreatAsAtomicUnit=on
  If Action Subsystem3 : Subsystem  TreatAsAtomicUnit=on
  Merge : Merge  Inputs=4
  Out1 : Outport
  wires:
  PrevLane/1 -> If/1
  In2/1 -> If Action Subsystem/1(In1), If/2
  In3/1 -> If/3, If Action Subsystem1/1(In1)
  In4/1 -> If Action Subsystem2/1(In1), If/4
  In5/1 -> If Action Subsystem3/1(In1), If/5
  If/1 -> If Action Subsystem/Action
  If/2 -> If Action Subsystem1/Action
  If/3 -> If Action Subsystem2/Action
  If/4 -> If Action Subsystem3/Action
  If Action Subsystem/1(Out1) -> Merge/1
  If Action Subsystem1/1(Out1) -> Merge/2
  If Action Subsystem2/1(Out1) -> Merge/3
  If Action Subsystem3/1(Out1) -> Merge/4
  Merge/1 -> Out1/1

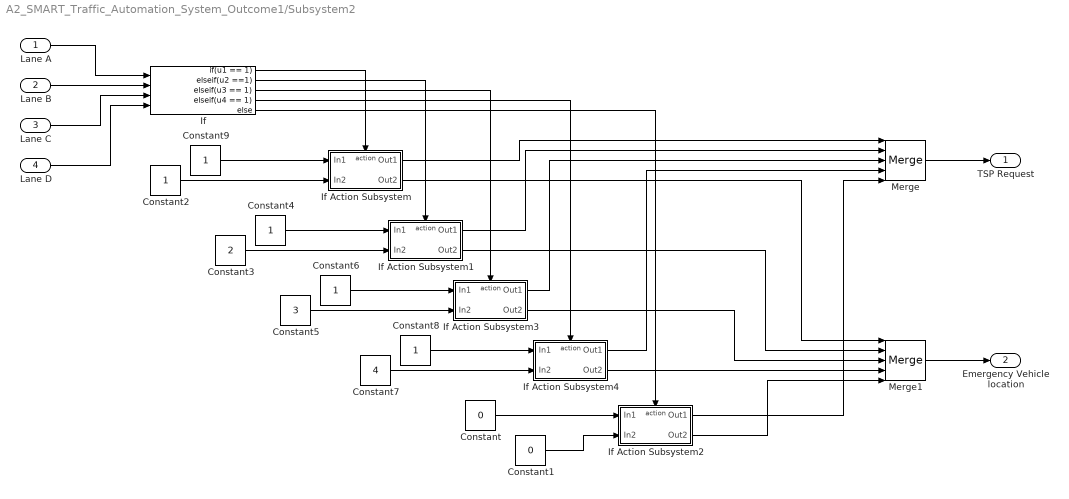
== system A2_SMART_Traffic_Automation_System_Outcome1/Subsystem2 ==
  Lane A : Inport
  Lane B : Inport  Port=2
  Lane C : Inport  Port=3
  Lane D : Inport  Port=4
  Constant : Constant  Value=0
  Constant1 : Constant  Value=0
  Constant{2,4,6,8..9} (5 alike) : Constant
  Constant3 : Constant  Value=2
  Constant5 : Constant  Value=3
  Constant7 : Constant  Value=4
  If : If  NumInputs=4  IfExpression=u1 == 1  ElseIfExpressions=u2 ==1, u3 == 1, u4 == 1
  If Action Subsystem : Subsystem  TreatAsAtomicUnit=on
  If Action Subsystem1 : Subsystem  TreatAsAtomicUnit=on
  If Action Subsystem2 : Subsystem  TreatAsAtomicUnit=on
  If Action Subsystem3 : Subsystem  TreatAsAtomicUnit=on
  If Action Subsystem4 : Subsystem  TreatAsAtomicUnit=on
  Merge : Merge  Inputs=5
  Merge1 : Merge  Inputs=5
  TSP Request : Outport
  Emergency Vehicle location : Outport  Port=2
  wires:
  If/2 -> If Action Subsystem1/Action
  If/1 -> If Action Subsystem/Action
  Constant9/1 -> If Action Subsystem/1(In1)
  Lane A/1 -> If/1
  Lane B/1 -> If/2
  Constant2/1 -> If Action Subsystem/2(In2)
  Lane C/1 -> If/3
  Lane D/1 -> If/4
  If/3 -> If Action Subsystem3/Action
  If/4 -> If Action Subsystem4/Action
  Merge1/1 -> Emergency Vehicle location/1
  Merge/1 -> TSP Request/1
  If Action Subsystem/1(Out1) -> Merge/1
  If Action Subsystem1/1(Out1) -> Merge/2
  If Action Subsystem3/1(Out1) -> Merge/3
  If Action Subsystem4/1(Out1) -> Merge/4
  Constant3/1 -> If Action Subsystem1/2(In2)
  Constant4/1 -> If Action Subsystem1/1(In1)
  Constant5/1 -> If Action Subsystem3/2(In2)
  Constant6/1 -> If Action Subsystem3/1(In1)
  Constant7/1 -> If Action Subsystem4/2(In2)
  Constant8/1 -> If Action Subsystem4/1(In1)
  If Action Subsystem/2(Out2) -> Merge1/1
  If Action Subsystem1/2(Out2) -> Merge1/2
  If Action Subsystem3/2(Out2) -> Merge1/3
  If Action Subsystem4/2(Out2) -> Merge1/4
  If/5 -> If Action Subsystem2/Action
  Constant/1 -> If Action Subsystem2/1(In1)
  Constant1/1 -> If Action Subsystem2/2(In2)
  If Action Subsystem2/1(Out1) -> Merge/5
  If Action Subsystem2/2(Out2) -> Merge1/5

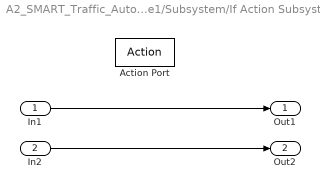
== system A2_SMART_Traffic_Automation_System_Outcome1/Subsystem/If Action Subsystem ==
  In1 : Inport
  In2 : Inport  Port=2
  Action Port : ActionPort  ActionPortLabel=if(u1 > 0)
  Out1 : Outport
  Out2 : Outport  Port=2
  wires:
  In1/1 -> Out1/1
  In2/1 -> Out2/1

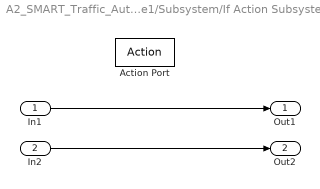
== system A2_SMART_Traffic_Automation_System_Outcome1/Subsystem/If Action Subsystem1 ==
  In1 : Inport
  In2 : Inport  Port=2
  Action Port : ActionPort  ActionPortLabel=elseif(u2 > 0)
  Out1 : Outport
  Out2 : Outport  Port=2
  wires:
  In1/1 -> Out1/1
  In2/1 -> Out2/1

== system A2_SMART_Traffic_Automation_System_Outcome1/Subsystem/If Action Subsystem2 ==
  In1 : Inport
  In2 : Inport  Port=2
  Action Port : ActionPort  ActionPortLabel=else
  Out1 : Outport
  Out2 : Outport  Port=2
  wires:
  In1/1 -> Out1/1
  In2/1 -> Out2/1

== system A2_SMART_Traffic_Automation_System_Outcome1/Subsystem1/If Action Subsystem ==
  In1 : Inport
  Action Port : ActionPort  ActionPortLabel=if(u1 == 4)
  Out1 : Outport
  wires:
  In1/1 -> Out1/1

== system A2_SMART_Traffic_Automation_System_Outcome1/Subsystem1/If Action Subsystem1 ==
  In1 : Inport
  Action Port : ActionPort  ActionPortLabel=elseif(u1 == 1)
  Out1 : Outport
  wires:
  In1/1 -> Out1/1

== system A2_SMART_Traffic_Automation_System_Outcome1/Subsystem1/If Action Subsystem2 ==
  In1 : Inport
  Action Port : ActionPort  ActionPortLabel=elseif( u1 == 2)
  Out1 : Outport
  wires:
  In1/1 -> Out1/1

== system A2_SMART_Traffic_Automation_System_Outcome1/Subsystem1/If Action Subsystem3 ==
  In1 : Inport
  Action Port : ActionPort  ActionPortLabel=elseif( u1 == 3)
  Out1 : Outport
  wires:
  In1/1 -> Out1/1

== system A2_SMART_Traffic_Automation_System_Outcome1/Subsystem2/If Action Subsystem ==
  In1 : Inport
  In2 : Inport  Port=2
  Action Port : ActionPort  ActionPortLabel=if(u1 == 1)
  Out1 : Outport
  Out2 : Outport  Port=2
  wires:
  In1/1 -> Out1/1
  In2/1 -> Out2/1

== system A2_SMART_Traffic_Automation_System_Outcome1/Subsystem2/If Action Subsystem1 ==
  In1 : Inport
  In2 : Inport  Port=2
  Action Port : ActionPort  ActionPortLabel=elseif(u2 ==1)
  Out1 : Outport
  Out2 : Outport  Port=2
  wires:
  In1/1 -> Out1/1
  In2/1 -> Out2/1

== system A2_SMART_Traffic_Automation_System_Outcome1/Subsystem2/If Action Subsystem2 ==
  In1 : Inport
  In2 : Inport  Port=2
  Action Port : ActionPort  ActionPortLabel=else
  Out1 : Outport
  Out2 : Outport  Port=2
  wires:
  In1/1 -> Out1/1
  In2/1 -> Out2/1

== system A2_SMART_Traffic_Automation_System_Outcome1/Subsystem2/If Action Subsystem3 ==
  In1 : Inport
  In2 : Inport  Port=2
  Action Port : ActionPort  ActionPortLabel=elseif( u3 == 1)
  Out1 : Outport
  Out2 : Outport  Port=2
  wires:
  In1/1 -> Out1/1
  In2/1 -> Out2/1

== system A2_SMART_Traffic_Automation_System_Outcome1/Subsystem2/If Action Subsystem4 ==
  In1 : Inport
  In2 : Inport  Port=2
  Action Port : ActionPort  ActionPortLabel=elseif( u4 == 1)
  Out1 : Outport
  Out2 : Outport  Port=2
  wires:
  In1/1 -> Out1/1
  In2/1 -> Out2/1

== stateflow chart A2_SMART_Traffic_Automation_System_Outcome1/Light Controller (A) ==
  settings: executeAtInitialization=1
  state Green
    S0=1;
    S1=0;
  state Amber
    S0=0;
    S1=1;
  state Red
    S0=0;
    S1=0;
  (default) -> Green
  Red -> Green : [Green==1]
  Green -> Amber : [Green==0]
  Amber -> Red : after(3, sec)
  data: Green input; S0 output; S1 output

== stateflow chart A2_SMART_Traffic_Automation_System_Outcome1/Light Controller (B) ==
  settings: executeAtInitialization=1
  state Green
    S0=1;
    S1=0;
  state Amber
    S0=0;
    S1=1;
  state Red
    S0=0;
    S1=0;
  Red -> Green : [Green==1]
  Green -> Amber : [Green==0]
  (default) -> Red
  Amber -> Red : after(3, sec)
  data: Green input; S0 output; S1 output

== stateflow chart A2_SMART_Traffic_Automation_System_Outcome1/Trafftc Controller ==
  settings: executeAtInitialization=1
  state Traffic_control
    state TSP [parallel]
      settings: executionOrder=2
      note: Signal adjustment based on:
          | Current Phase
          | Current Lane At
          | Arrival Time
          | Crossing Time
      note: TSP Request Received
      note: Green Extension (Only Emergency Vehicle)
      state No_Signal_Alteration
        Extend_s=0;
        % No need green extension
      state No_Request
        Terminate_s=-1;
        Extend_s=0;
        TSP_ART=0;
        TSP_Emergency=0;
        % Initialize
      state Green_Extension
        Extend_s=MaxGreenExt;
        % Maximum Green Extension granted
        % Arrival Time + Crossing Time must smaller than 20s
        % vehicle should operate at speed above 35 km/h
      state ART_Interupt_EmergencyVehicleTSP
        Terminate_s=-1;
        Extend_s=0;
        % Initialize
      note: Early Green Call
      state EarlyGreen_1
        Terminate_s=max(MinGreen,t+ArrivalTime-6);
        % Current phase will terminate earlier
        % Terminate_s is the maximum allowed green interval
        % Phase should terminate 6s (3s amber and 3s red) before arrival
        % ArrivalTime - 6 should be less than or equal than 15s (green interval)
        % For arrival time less than 21s, vehicle should operates at speed above 31km/h
        % Also considering arrival time >= Minimum green (2s) + amber + red = 8s
        % Speed is limited to be below 81 km/h
      state TSP_Emergency
        TSP_Emergency=1;
        % Wait for current phase end
        % and enter hold state
      state TSP_ART
        % Wait for current phase end
        % and enter hold state
      state EarlyGreen_2
        Terminate_s=max(MinGreen,ArrivalTime-8);
        % One more phase is allowed with maximum possible green time
        % For emergency vehicle preemption,
        % after this phase, phase insertion is introduced.
      note: TSP For ART
      state ART_Crossing
        TSP_ART=1;
        % remain in hold state whil e ART crossing
      note: Insert one more phase before TSP granted
      state Phase_Skipping_A
        Lane=1;
        % Skip to Lane B
        % In hold state, upcoming green lane will be
        %the next lane of  'Lane'
      state One_More_Phase
        TSP_Emergency=1;
      note: TSP For Emergency Vehicle
      state Phase_Skipping
        Lane=At;
        % Skip to the next lane
        % of emergency vehicle currently at
      state No_Memory_needed
        TSP_ART=0;
        TSP_Emergency=0;
        Terminate_s=-1;
      state Memory_B
        Lane=mod(At-2,4) + 1;
        TSP_ART=0;
        TSP_Emergency=1;
        Terminate_s=-1;
        % Serve upcoming lane as
        %at the lane emergency vehicle at
      state Memory_C
        Lane=mod(At-2,4) + 1;
        TSP_ART=0;
        TSP_Emergency=1;
        Terminate_s=-1;
        % Serve upcoming lane as
        %at the lane emergency vehicle at
      state Memory_D
        Lane=mod(At-2,4) + 1;
        TSP_ART=0;
        TSP_Emergency=1;
        Terminate_s=-1;
        % Serve upcoming lane as
        %at the lane emergency vehicle at
      state ART_Interupt
        TSP_Emergency=1;
      state Memory_A
        Lane=mod(At-2,4) + 1;
        TSP_ART=0;
        TSP_Emergency=1;
        Terminate_s=-1;
        % Serve upcoming lane as
        %at the lane emergency vehicle at
      state Green_State2
      state Green_State
      state Green_State1
      state Green_State3
      state Resume_Cycle_B
        Lane=1;
      state Resume_Cycle_C
        Lane=2;
      state Resume_Cycle_D
        Lane=3;
      state Resume_Cycle_A
        Lane=4;
      note: Memory for Upcoming Phase after TSP granted
      (junction 960) -> No_Request
      (junction 522) -> No_Request : [Emergency==0 || t>GreenInterval+Extend_s]
      TSP_Emergency -> ART_Interupt_EmergencyVehicleTSP [order 1] : % If ART Request present suddenly
          | [ART==1]
      (default) -> No_Request
      No_Request -> (junction 566) : % If transit request received
          | [ART==1 || Emergency==1]
      (junction 566) -> (junction 532) [order 1] : % If no ART Transit Request
          | % AND
          | % If current phase is the lane where Emergency Vechicle at
          | % AND
          | % is in green interval
          | [ART==0 && ...
          | Lane==At && Hold==0]
      No_Signal_Alteration -> (junction 522)
      (junction 532) -> No_Signal_Alteration [order 1] : % If Emergency Vehicle can finish crossing within Green Interval
          | [ArrivalTime+CrossingTime<GreenInterval-t]
      ART_Interupt_EmergencyVehicleTSP -> (junction 566)
      (junction 566) -> (junction 533) [order 2]
      (junction 532) -> Green_Extension [order 2]
      Green_Extension -> (junction 522)
      (junction 509) -> No_Request
      (junction 938) -> ART_Interupt_EmergencyVehicleTSP
      ART_Crossing -> (junction 960) [order 2] : % ART cancel transit request
          | [ART==0]
      EarlyGreen_1 -> TSP_Emergency [order 2] : [Emergency==1]
      (junction 533) -> EarlyGreen_1 [order 1] : % If current phase is GREEN
          | [Hold==0]
      (junction 533) -> (junction 386) [order 2]
      EarlyGreen_1 -> TSP_ART [order 1] : [ART==1]
      TSP_Emergency -> (junction 955) [order 2]
      (junction 386) -> (junction 433) [order 2] : % One more phase is not allowed
      (junction 386) -> EarlyGreen_2 [order 1] : % If one more phase is allowed
          | [ArrivalTime>=8+6-t]
      TSP_ART -> (junction 955)
      EarlyGreen_2 -> (junction 451) [order 2]
      EarlyGreen_2 -> (junction 560) [order 1] : [Hold==0 && ART==1]
      (junction 955) -> (junction 433) : % After green state end and enter hold state
          | [Hold==1]
      (junction 433) -> ART_Crossing [order 1] : [ART==1]
      (junction 433) -> (junction 982) [order 2]
      One_More_Phase -> (junction 433) : % Back to hold state
          | [Hold==1]
      (junction 560) -> ART_Crossing : % after one more phase is ended
          | [t>Terminate_s]
      ART_Crossing -> (junction 500) [order 1] : % ART interrupt emergency vehicle TSP,
          | % after ART finish crossing, emergency vehicle hasn't finish crossing
          | [ART==0 && TSP_Emergency==1 && Emergency==1]
      (junction 451) -> (junction 530) [order 1] : % If upcoming green lane is the lane where emergency vehicle at
          | [Lane == mod(At-2,4) + 1]
      (junction 451) -> One_More_Phase [order 2] : % Upcoming lane is not the lane where emergency at
          | [Hold==0]
      (junction 982) -> (junction 500) [order 1] : % If upcoming green lane is not lane where emergency vehicle at
          | [Lane ~= (mod(At-2,4) + 1)]
      (junction 982) -> No_Memory_needed [order 2] : % upcoming green lane is the lane where emergency vehicle at
          | % therefore, no signal alteration
          | [TSP_Emergency==1 && Lane == (mod(At-2,4) + 1)]
      (junction 530) -> Phase_Skipping_A [order 1] : [Lane==4]
      (junction 530) -> Phase_Skipping [order 2]
      Phase_Skipping_A -> One_More_Phase : [Hold==0]
      Phase_Skipping -> One_More_Phase : [Hold==0]
      (junction 500) -> Memory_A [order 1] : [Lane==4]
      (junction 500) -> Memory_B [order 4] : [Lane==1]
      (junction 500) -> Memory_D [order 2] : [Lane==3]
      (junction 500) -> Memory_C [order 3] : [Lane==2]
      No_Memory_needed -> ART_Interupt [order 1] : [ART==1]
      No_Memory_needed -> (junction 509) [order 2] : [Emergency==0]
      Memory_B -> (junction 1012) [order 1] : [ART==1]
      Memory_B -> Green_State [order 2] : % Back to green state
          | [Hold==0]
      Memory_C -> (junction 1012) [order 1] : [ART==1]
      Memory_C -> Green_State1 [order 2] : % Back to green state
          | [Hold==0]
      ART_Interupt -> (junction 938)
      Memory_D -> (junction 1012) [order 1] : [ART==1]
      Green_State2 -> (junction 1012) [order 1] : [ART==1]
      Green_State3 -> (junction 1012) [order 1] : [ART==1]
      Memory_A -> (junction 1012) [order 1] : [ART==1]
      (junction 1012) -> (junction 938) : %  If ART Request present suddenly
      Green_State1 -> (junction 1012) [order 1] : [ART==1]
      Green_State -> (junction 1012) [order 1] : [ART==1]
      Memory_D -> Green_State2 [order 2] : % Back to green state
          | [Hold==0]
      Memory_A -> Green_State3 [order 2] : % Back to green state
          | [Hold==0]
      Green_State2 -> Resume_Cycle_D [order 2] : % Back to hold state
          | [Hold==1]
      Green_State -> Resume_Cycle_B [order 2] : % Back to hold state
          | [Hold==1]
      Green_State1 -> Resume_Cycle_C [order 2] : % Back to hold state
          | [Hold==1]
      Green_State3 -> Resume_Cycle_A [order 2] : % Back to hold state
          | [Hold==1]
      Resume_Cycle_B -> (junction 509)
      Resume_Cycle_C -> (junction 509)
      Resume_Cycle_D -> (junction 509)
      Resume_Cycle_A -> (junction 509)
    state TrafficLight_Transition [parallel]
      settings: executionOrder=1
      state LaneD
        A=0;
        B=0;
        C=0;
        D=1;
        t=temporalCount(sec);
        Hold=0;
        Lane=4;
      state LaneA
        A=1;
        B=0;
        C=0;
        D=0;
        t=temporalCount(sec);
        Hold=0;
        Lane=1;
      state Hold
        A=0;
        B=0;
        C=0;
        D=0;
        t=temporalCount(sec);
        Hold=1;
        PrevLane=Lane;
      state LaneB
        A=0;
        B=1;
        C=0;
        D=0;
        t=temporalCount(sec);
        Hold=0;
        Lane=2;
      state LaneC
        A=0;
        B=0;
        C=1;
        D=0;
        t=temporalCount(sec);
        Hold=0;
        Lane=3;
      (default) -> LaneA
      Hold -> LaneD [order 3] : [Lane==3 && t>6]
      LaneA -> Hold : % Green Interval for normal operation end OR
          | % Phase should terminates earlier to reserve TSP OR
          | % Emergency vehicle cancel transit request
          | [t >= GreenInterval+Extend_s || ...
          | (t>Terminate_s && Terminate_s>-1) || ...
          | (TSP_Emergency==1 && Emergency==0)]
      Hold -> Hold [order 1] : % ART Crossing
          | [TSP_ART == 1]
      LaneD -> Hold : % Green Interval for normal operation end OR
          | % Phase should terminates earlier to reserve TSP OR
          | % Emergency vehicle cancel transit request
          | [t >= GreenInterval+Extend_s || ...
          | (t>Terminate_s && Terminate_s>-1) || ...
          | (TSP_Emergency==1 && Emergency==0)]
      Hold -> LaneA [order 2] : [Lane==4 && t>6]
      Hold -> LaneC [order 5] : [Lane==2 && t>6]
      LaneB -> Hold : % Green Interval for normal operation end OR
          | % Phase should terminates earlier to reserve TSP OR
          | % Emergency vehicle cancel transit request
          | [t >= GreenInterval+Extend_s || ...
          | (t>Terminate_s && Terminate_s>-1) || ...
          | (TSP_Emergency==1 && Emergency==0)]
      Hold -> LaneB [order 4] : [Lane==1 && t>6]
      LaneC -> Hold : % Green Interval for normal operation end OR
          | % Phase should terminates earlier to reserve TSP OR
          | % Emergency vehicle cancel transit request
          | [t >= GreenInterval+Extend_s || ...
          | (t>Terminate_s && Terminate_s>-1) || ...
          | (TSP_Emergency==1 && Emergency==0)]
    state Flash [parallel]
      settings: executionOrder=3
      state Not_Flash
        Flash=0;
      state Flash_1
        Flash=1;
      state Flash_2
        Flash=0;
      (default) -> Not_Flash
      Flash_1 -> Not_Flash [order 1] : [ART==0]
      Not_Flash -> Flash_1 : % If TSP is reserved for ART
          | [TSP_ART==1 && ART==1]
      Flash_1 -> Flash_2 [order 2] : after(0.2, sec)
      Flash_2 -> Flash_1 : after(0.2, sec)
  (default) -> Traffic_control
  data: GreenInterval input =15; A output; B output; C output; D output; t local =0; Hold local =0; ArrivalTime input; CrossingTime input; ART input; MaxGreenExt local =20; MinGreen local =2; Terminate_s local =0; Extend_s local =0; Flash output; Lane local =2; Emergency input; At input; PrevLane output =4; TSP_ART local =0; TSP_Emergency local =0

== stateflow chart A2_SMART_Traffic_Automation_System_Outcome1/Light Controller (C) ==
  settings: executeAtInitialization=1
  state Green
    S0=1;
    S1=0;
  state Amber
    S0=0;
    S1=1;
  state Red
    S0=0;
    S1=0;
  Red -> Green : [Green==1]
  Green -> Amber : [Green==0]
  (default) -> Red
  Amber -> Red : after(3, sec)
  data: Green input; S0 output; S1 output

== stateflow chart A2_SMART_Traffic_Automation_System_Outcome1/Light Controller (D) ==
  settings: executeAtInitialization=1
  state Green
    S0=1;
    S1=0;
  state Amber
    S0=0;
    S1=1;
  state Red
    S0=0;
    S1=0;
  Red -> Green : [Green==1]
  Green -> Amber : [Green==0]
  (default) -> Red
  Amber -> Red : after(3, sec)
  data: Green input; S0 output; S1 output

== stateflow chart A2_SMART_Traffic_Automation_System_Outcome1/Chart ==
  state TSP_Not_Received
  state TSP_ART
    ArrivalTime=ArrivalTime_ART;
    CrossingTime=CrossingTime_ART;
    At=At_ART;
  state TSP_EmergencyVehicle
    ArrivalTime=ArrivalTime_Emergency;
    CrossingTime=CrossingTime_Emergency;
    At=At_Emergency;
  (default) -> TSP_Not_Received
  TSP_Not_Received -> TSP_ART [order 1] : [ART==1]
  TSP_EmergencyVehicle -> TSP_ART [order 1] : [ART==1]
  (junction 10) -> TSP_Not_Received [order 2]
  TSP_EmergencyVehicle -> TSP_Not_Received [order 2] : [Emergency==0]
  TSP_Not_Received -> TSP_EmergencyVehicle [order 2] : [Emergency==1]
  TSP_ART -> (junction 10) : [ART==0]
  (junction 10) -> TSP_EmergencyVehicle [order 1] : [Emergency==1]
  data: ArrivalTime_ART input; ArrivalTime_Emergency input; CrossingTime_ART input; CrossingTime_Emergency input; Emergency input; ArrivalTime output =0; CrossingTime output =0; ART input; At output =0; At_Emergency input; At_ART input

== stateflow chart A2_SMART_Traffic_Automation_System_Outcome1/Chart2 ==
  state No_or_Cancel_Request
    Emergency=0;
    Arrived=0;
  state Request_received
    Emergency=1;
  state ART_Arrived
    Emergency=1;
    Arrived=1;
  (default) -> No_or_Cancel_Request
  No_or_Cancel_Request -> Request_received : [TSP==1]
  ART_Arrived -> No_or_Cancel_Request : [TSP==0]
  Request_received -> ART_Arrived : after(ArrivalTime,sec)
  data: TSP input; ArrivalTime input; Arrived output; Emergency output

== stateflow chart A2_SMART_Traffic_Automation_System_Outcome1/Traffic Congestion Determination ==
  settings: stateMachineType=MOORE_MACHINE  executeAtInitialization=1
  state Low_Traffic
    GreenInterval=15;
  state Medium_Traffic1
    GreenInterval=30;
  state Empty_Traffic
    GreenInterval=3;
  state High_Traffic
    GreenInterval=45;
  Empty_Traffic -> Medium_Traffic1 [order 3] : [Medium==1]
  (default) -> Low_Traffic
  Low_Traffic -> Medium_Traffic1 [order 1] : [Medium==1]
  Medium_Traffic1 -> Empty_Traffic [order 3] : [Low==0 && Medium==0 && High==0]
  Medium_Traffic1 -> Low_Traffic [order 1] : [Low==1]
  High_Traffic -> Medium_Traffic1 [order 1] : [Medium==1]
  Medium_Traffic1 -> High_Traffic [order 2] : [High==1]
  Empty_Traffic -> Low_Traffic [order 1] : [Low==1]
  Low_Traffic -> Empty_Traffic [order 3] : [Low==0 && Medium==0 && High==0]
  High_Traffic -> Low_Traffic [order 2] : [Low==1]
  Low_Traffic -> High_Traffic [order 2] : [High==1]
  Empty_Traffic -> High_Traffic [order 2] : [High==1]
  High_Traffic -> Empty_Traffic [order 3] : [Low==0 && Medium==0 && High==0]
  data: Low input; Medium input; High input; GreenInterval output

== stateflow chart A2_SMART_Traffic_Automation_System_Outcome1/Chart1 ==
  state No_or_Cancel_Request
    ART=0;
    Arrived=0;
  state Request_received
    ART=1;
  state ART_Arrived
    ART=1;
    Arrived=1;
  (default) -> No_or_Cancel_Request
  No_or_Cancel_Request -> Request_received : [TSP==1]
  ART_Arrived -> No_or_Cancel_Request [order 2] : [TSP==0]
  ART_Arrived -> No_or_Cancel_Request [order 1] : after(CrossingTime,sec)
  Request_received -> ART_Arrived : after(ArrivalTime,sec)
  data: TSP input; ArrivalTime input; CrossingTime input; ART output; Arrived output
